simulink model "sampleModel106"  (R2022a)
settings: Solver=VariableStepAuto  StartTime=0.0  StopTime=10.0  RelTol=1e-3
undefined symbols (not defined in the file): DiscIntNeverNeededParam, magnitude, Newton, Raphson
libraries: simulink x379, slpidlib x89
(part 2 of 16)

== system sampleModel106/cfblk78/cfblk12 ==
  cfblk1 : Inport
  cfblk6 : Inport  Port=2
  Action Port : ActionPort  ActionPortLabel=else
  cfblk3 : ComplexToMagnitudeAngle
  cfblk4 : Subsystem
  cfblk5 : Subsystem
  cfblk8 : Delay
  cfblk9 : Delay
  cfblk2 : Outport
  cfblk7 : Outport  Port=2
  wires:
  cfblk6/1 -> cfblk5/1(cfblk1)
  cfblk1/1 -> cfblk3/1
  cfblk4/1(cfblk2) -> cfblk5/2(cfblk11)
  cfblk4/2(cfblk14) -> cfblk2/1
  cfblk5/3(cfblk13) -> cfblk7/1
  cfblk3/1 -> cfblk4/3(cfblk12)
  cfblk3/2 -> cfblk4/4(cfblk13)
  cfblk5/1(cfblk2) -> cfblk8/1
  cfblk8/1 -> cfblk4/1(cfblk1)
  cfblk5/2(cfblk12) -> cfblk9/1
  cfblk9/1 -> cfblk4/2(cfblk11)

== system sampleModel106/cfblk79/cfblk6 ==
  cfblk1 : Inport
  cfblk10 : Delay  SampleTime=1
  cfblk3 : Product
  cfblk4 : Squeeze
  cfblk5 : Product
  cfblk6 : Constant  Value=[-50724463.125212]  SampleTime=1
  cfblk7 : Constant  Value=[-745768619.596792]  SampleTime=1
  cfblk8 : Subsystem
  cfblk9 : Delay  SampleTime=1
  cfblk2 : Outport
  wires:
  cfblk4/1 -> cfblk2/1
  cfblk6/1 -> cfblk4/1
  cfblk7/1 -> cfblk3/1
  cfblk1/1 -> cfblk8/1(cfblk1)
  cfblk8/1(cfblk2) -> cfblk5/1
  cfblk8/2(cfblk9) -> cfblk3/2, cfblk5/2
  cfblk5/1 -> cfblk9/1
  cfblk9/1 -> cfblk8/3(cfblk8)
  cfblk3/1 -> cfblk10/1
  cfblk10/1 -> cfblk8/2(cfblk7)

== system sampleModel106/cfblk79/cfblk7 ==
  cfblk1 : Inport
  cfblk14 : Inport  Port=2
  cfblk15 : Inport  Port=3
  cfblk10 : Subsystem
  cfblk11 : Subsystem
  cfblk12 : Subsystem
  cfblk13 : Subsystem
  cfblk16 : Delay  SampleTime=1
  cfblk17 : Delay  SampleTime=1
  cfblk3 : DiscreteStateSpace
  cfblk4 : DiscreteZeroPole  Poles=[0 0.5]  Gain=1
  cfblk5 : simulink/Discrete/Tapped Delay  vinit=0.0  samptime=-1  NumDelays=1  DelayOrder=Oldest  includeCurrent=off
  cfblk6 : simulink/Math Operations/MinMax Running Resettable  Function=min  vinit=0.0
  cfblk7 : simulink/Math Operations/MinMax Running Resettable  Function=min  vinit=0.0
  cfblk8 : Constant  Value=[66779856.754441]  SampleTime=1
  cfblk9 : Constant  Value=[74672410.841103]  SampleTime=1
  cfblk2 : Outport
  wires:
  cfblk15/1 -> cfblk7/1
  cfblk11/1(cfblk2) -> cfblk5/1
  cfblk5/1 -> cfblk3/1
  cfblk13/1(cfblk2) -> cfblk2/1
  cfblk7/1 -> cfblk13/1(cfblk1)
  cfblk3/1 -> cfblk10/1(cfblk1)
  cfblk8/1 -> cfblk11/1(cfblk1)
  cfblk4/1 -> cfblk12/1(cfblk1)
  cfblk10/1(cfblk2) -> cfblk7/2
  cfblk1/1 -> cfblk6/2
  cfblk9/1 -> cfblk12/2(cfblk15)
  cfblk6/1 -> cfblk11/2(cfblk13)
  cfblk11/3(cfblk16) -> cfblk12/3(cfblk16)
  cfblk14/1 -> cfblk4/1
  cfblk11/2(cfblk15) -> cfblk16/1
  cfblk16/1 -> cfblk6/1
  cfblk12/1(cfblk2) -> cfblk17/1
  cfblk17/1 -> cfblk11/3(cfblk14)

== system sampleModel106/cfblk79/cfblk8 ==
  cfblk1 : Inport
  cfblk10 : Subsystem
  cfblk11 : Subsystem
  cfblk12 : Delay  SampleTime=1
  cfblk13 : Delay  SampleTime=1
  cfblk14 : Delay  SampleTime=1
  cfblk3 : Delay  DelayLengthSource=Input port  SampleTime=1
      settings: InputPortMap=u0,p1
  cfblk4 : slpidlib/PID Controller (2DOF)  Controller=PID  Form=Parallel  TimeDomain=Discrete-time  UseExternalTs=off  SampleTime=1  IntegratorMethod=Forward Euler  FilterMethod=Forward Euler  ControllerParametersSource=internal  P=1  I=1  UseKiTs=off  D=0  N=100  UseFilter=on  b=1  c=1  TunerSelectOption=Transfer Function Based (PID Tuner App)  InitialConditionSource=internal  InitialConditionForIntegrator=0  InitialConditionForFilter=0  DifferentiatorICPrevScaledInput=0  ExternalReset=none  TrackingMode=off  Kt=1  LimitOutput=off  SatLimitsSource=internal  UpperSaturationLimit=inf  LowerSaturationLimit=-inf  LinearizeAsGain=off  AntiWindupMode=none  Kb=1  POutMin=[]  POutMax=[]  IOutMin=[]  IOutMax=[]  DOutMin=[]  DOutMax=[]  NOutMin=[]  NOutMax=[]  bOutMin=[]  bOutMax=[]  cOutMin=[]  cOutMax=[]  SumOutMin=[]  SumOutMax=[]  SaturationOutMin=[]  SaturationOutMax=[]  PParamMin=[]  PParamMax=[]  IParamMin=[]  IParamMax=[]  DParamMin=[]  DParamMax=[]  NParamMin=[]  NParamMax=[]  bParamMin=[]  bParamMax=[]  cParamMin=[]  cParamMax=[]  KbParamMin=[]  KbParamMax=[]  KtParamMin=[]  KtParamMax=[]  KbOutMin=[]  KbOutMax=[]  KtOutMin=[]  KtOutMax=[]  IntegratorOutMin=[]  IntegratorOutMax=[]  FilterOutMin=[]  FilterOutMax=[]  SumI1OutMin=[]  SumI1OutMax=[]  SumI2OutMin=[]  SumI2OutMax=[]  SumI3OutMin=[]  SumI3OutMax=[]  SumI4OutMin=[]  SumI4OutMax=[]  SumDOutMin=[]  SumDOutMax=[]  Sum1OutMin=[]  Sum1OutMax=[]  Sum2OutMin=[]  Sum2OutMax=[]  Sum3OutMin=[]  Sum3OutMax=[]  DifferentiatorOutMin=[]  DifferentiatorOutMax=[]  FilterDiffOutCoefMin=[]  FilterDiffOutCoefMax=[]  ReciprocalOutMin=[]  ReciprocalOutMax=[]  SumDenOutMin=[]  SumDenOutMax=[]  SumNumOutMin=[]  SumNumOutMax=[]  DivideOutMin=[]  DivideOutMax=[]  UdiffTsProdOutMin=[]  UdiffTsProdOutMax=[]  NTsProdOutMin=[]  NTsProdOutMax=[]  UintegralTsProdOutMin=[]  UintegralTsProdOutMax=[]  UngainTsProdOutMin=[]  UngainTsProdOutMax=[]  IntegratorContinuousStateAttributes=''  IntegratorStateMustResolveToSignalObject=off  IntegratorRTWStateStorageClass=Auto  FilterContinuousStateAttributes=''  FilterStateMustResolveToSignalObject=off  FilterRTWStateStorageClass=Auto  ParallelPVariant=InternalParameters  IdealPVariant=Disabled  IVariant=InternalParameters  DVariant=InternalParameters  bVariant=InternalParameters  cVariant=InternalParameters  IntegratorVariant=Discrete  SatVariant=Disabled  AWVariant=Passthrough  PCopyVariant=Disabled  TRVariant=Disabled  FdbkBlocksVariant=Forward  IdealPFdbkVariant=Disabled  SatFdbkVariant=Disabled  DerivativeFilterVariant=ForwardEulerFilter  NVariant=InternalParameters  NCopyVariant=Disabled  FilterICVariant=InternalICsFilter  IntegratorICVariant=InternalICs  ExternalResetVariant=Disabled  TRSumVariant=Passthrough  SumFdbkVariant=Disabled  SumVariant=Sum_PID  TsampFilterVariant=InternalTs  TsampNgainVariant=Passthrough  TsampIntegralVariant=Passthrough  ExternalSaturationOutDataTypeStr=Inherit: Same as second input
      settings: SourceProductBaseCode=SL
  cfblk5 : DotProduct  OutDataTypeStr=Inherit: Inherit via internal rule
  cfblk6 : UnaryMinus
  cfblk7 : Constant  Value=[335459876.911431]  SampleTime=1
  cfblk8 : Constant  Value=[-968015926.513109]  SampleTime=1
  cfblk9 : Subsystem
  cfblk2 : Outport
  wires:
  cfblk8/1 -> cfblk10/1(cfblk1)
  cfblk10/1(cfblk2) -> cfblk6/1
  cfblk10/2(cfblk9) -> cfblk3/2
  cfblk9/1(cfblk2) -> cfblk11/1(cfblk1)
  cfblk11/1(cfblk2) -> cfblk4/1
  cfblk7/1 -> cfblk4/2
  cfblk1/1 -> cfblk2/1
  cfblk11/2(cfblk15) -> cfblk5/1
  cfblk6/1 -> cfblk9/1(cfblk1)
  cfblk10/3(cfblk10) -> cfblk5/2, cfblk11/2(cfblk14)
  cfblk3/1 -> cfblk9/3(cfblk11)
  cfblk4/1 -> cfblk12/1
  cfblk12/1 -> cfblk9/2(cfblk10)
  cfblk5/1 -> cfblk13/1
  cfblk13/1 -> cfblk3/1
  cfblk11/3(cfblk16) -> cfblk14/1
  cfblk14/1 -> cfblk9/4(cfblk12)

== system sampleModel106/cfblk80/cfblk10 ==
  cfblk1 : Inport
  cfblk14 : Inport  Port=2
  cfblk15 : Inport  Port=3
  cfblk10 : Subsystem
  cfblk11 : Subsystem
  cfblk12 : Subsystem
  cfblk13 : If  IfExpression=u1 >= 0  SampleTime=1
  cfblk16 : Subsystem  TreatAsAtomicUnit=on
  cfblk17 : Subsystem  TreatAsAtomicUnit=on
  cfblk18 : Delay  SampleTime=1
  cfblk19 : Delay  SampleTime=1
  cfblk3 : UnitDelay  HasFrameUpgradeWarning=on
  cfblk4 : Math  Operator=transpose
  cfblk5 : Product
  cfblk6 : Signum
  cfblk7 : Subsystem
  cfblk8 : Subsystem
  cfblk9 : Subsystem
  cfblk2 : Outport
  wires:
  cfblk3/1 -> cfblk4/1
  cfblk14/1 -> cfblk10/1(cfblk1), cfblk8/1(cfblk1), cfblk17/2(cfblk16)
  cfblk1/1 -> cfblk10/2(cfblk13)
  cfblk8/1(cfblk2) -> cfblk7/1(cfblk1)
  cfblk7/1(cfblk2) -> cfblk13/1
  cfblk5/1 -> cfblk11/1(cfblk1)
  cfblk17/1(cfblk2) -> cfblk12/1(cfblk1)
  cfblk17/2(cfblk17) -> cfblk3/1
  cfblk10/1(cfblk2) -> cfblk9/2(cfblk10)
  cfblk12/1(cfblk2) -> cfblk5/1
  cfblk12/2(cfblk10) -> cfblk6/1
  cfblk16/1(cfblk2) -> cfblk5/2
  cfblk12/3(cfblk11) -> cfblk11/2(cfblk15)
  cfblk6/1 -> cfblk2/1
  cfblk15/1 -> cfblk9/3(cfblk11)
  cfblk9/1(cfblk2) -> cfblk16/2(cfblk7)
  cfblk10/2(cfblk14) -> cfblk17/1(cfblk1)
  cfblk13/1 -> cfblk16/Action
  cfblk13/2 -> cfblk17/Action
  cfblk11/1(cfblk2) -> cfblk18/1
  cfblk18/1 -> cfblk9/1(cfblk1)
  cfblk4/1 -> cfblk19/1
  cfblk19/1 -> cfblk16/1(cfblk1)

== system sampleModel106/cfblk80/cfblk11 ==
  cfblk1 : Inport
  cfblk11 : Inport  Port=2
  cfblk12 : Inport  Port=3
  cfblk10 : Subsystem
  cfblk15 : Delay  SampleTime=1
  cfblk16 : Delay  SampleTime=1
  cfblk3 : UnitDelay  HasFrameUpgradeWarning=on
  cfblk4 : UnitDelay  HasFrameUpgradeWarning=on
  cfblk5 : Delay  DelayLengthSource=Input port  SampleTime=1
      settings: InputPortMap=u0,p1
  cfblk6 : Abs  SaturateOnIntegerOverflow=off
  cfblk7 : Abs  SaturateOnIntegerOverflow=off
  cfblk8 : Subsystem
  cfblk9 : Subsystem
  cfblk2 : Outport
  cfblk13 : Outport  Port=2
  cfblk14 : Outport  Port=3
  wires:
  cfblk7/1 -> cfblk4/1
  cfblk10/1(cfblk2) -> cfblk3/1, cfblk8/4(cfblk15)
  cfblk11/1 -> cfblk13/1, cfblk9/3(cfblk15)
  cfblk12/1 -> cfblk2/1
  cfblk1/1 -> cfblk9/1(cfblk1)
  cfblk4/1 -> cfblk8/1(cfblk1)
  cfblk3/1 -> cfblk7/1
  cfblk9/1(cfblk2) -> cfblk6/1
  cfblk6/1 -> cfblk14/1
  cfblk5/1 -> cfblk8/2(cfblk13), cfblk15/1
  cfblk9/2(cfblk16) -> cfblk5/2
  cfblk9/3(cfblk17) -> cfblk10/1(cfblk1), cfblk8/3(cfblk14)
  cfblk15/1 -> cfblk9/2(cfblk14)
  cfblk8/1(cfblk2) -> cfblk16/1
  cfblk16/1 -> cfblk5/1

== system sampleModel106/cfblk80/cfblk12 ==
  cfblk1 : Inport
  cfblk10 : Inport  Port=2
  cfblk11 : Inport  Port=3
  cfblk13 : Delay  SampleTime=1
  cfblk3 : simulink/Math Operations/MinMax Running Resettable  Function=min  vinit=0.0
  cfblk4 : simulink/Math Operations/MinMax Running Resettable  Function=min  vinit=0.0
  cfblk5 : Constant  Value=[977677055.590889]  SampleTime=1
  cfblk6 : Constant  Value=[-64225626.397108]  SampleTime=1
  cfblk7 : Constant  Value=[-755451288.420639]  SampleTime=1
  cfblk8 : Constant  Value=[-818937205.633430]  SampleTime=1
  cfblk9 : Subsystem
  cfblk2 : Outport
  cfblk12 : Outport  Port=2
  wires:
  cfblk5/1 -> cfblk12/1
  cfblk10/1 -> cfblk3/1
  cfblk1/1 -> cfblk2/1
  cfblk4/1 -> cfblk9/1(cfblk1)
  cfblk11/1 -> cfblk3/2
  cfblk8/1 -> cfblk4/2
  cfblk9/1(cfblk2) -> cfblk13/1
  cfblk13/1 -> cfblk4/1

== system sampleModel106/cfblk80/cfblk8 ==
  cfblk1 : Inport
  cfblk9 : Inport  Port=2
  cfblk10 : Inport  Port=3
  cfblk11 : Inport  Port=4
  cfblk3 : simulink/Discrete/Transfer Fcn First Order  PoleZ=0.95  ICPrevOutput=0.0  DoSatur=off
  cfblk4 : Constant  Value=[816794916.066360]  SampleTime=1
  cfblk5 : Constant  Value=[815613005.147232]  SampleTime=1
  cfblk6 : Constant  Value=[-885196451.033393]  SampleTime=1
  cfblk7 : Subsystem
  cfblk8 : Subsystem
  cfblk2 : Outport
  wires:
  cfblk5/1 -> cfblk3/1
  cfblk6/1 -> cfblk7/1(cfblk1)
  cfblk1/1 -> cfblk7/2(cfblk7)
  cfblk10/1 -> cfblk2/1
  cfblk9/1 -> cfblk8/1(cfblk1)

== system sampleModel106/cfblk80/cfblk9 ==
  cfblk1 : Inport
  cfblk8 : Inport  Port=2
  cfblk11 : Subsystem  TreatAsAtomicUnit=on
  cfblk12 : Subsystem  TreatAsAtomicUnit=on
  cfblk13 : Delay  SampleTime=1
  cfblk3 : simulink/Discrete/Transfer Fcn Real Zero  ZeroZ=0.75  ICPrevInput=0.0  DoSatur=off
      settings: SourceProductBaseCode=SL
  cfblk4 : Trigonometry
  cfblk5 : Sin  TimeSource=Use external signal  SampleTime=0
  cfblk6 : Subsystem
  cfblk7 : If  IfExpression=u1 >= 0  SampleTime=1
  cfblk2 : Outport
  cfblk9 : Outport  Port=2
  cfblk10 : Outport  Port=3
  wires:
  cfblk5/1 -> cfblk3/1, cfblk9/1
  cfblk11/1(cfblk2) -> cfblk6/1(cfblk1)
  cfblk1/1 -> cfblk7/1, cfblk5/1
  cfblk12/1(cfblk2) -> cfblk6/2(cfblk15)
  cfblk8/1 -> cfblk6/3(cfblk16)
  cfblk11/2(cfblk11) -> cfblk12/1(cfblk1)
  cfblk6/1(cfblk2) -> cfblk2/1, cfblk13/1
  cfblk3/1 -> cfblk4/1
  cfblk4/1 -> cfblk10/1, cfblk11/1(cfblk1)
  cfblk7/1 -> cfblk11/Action
  cfblk7/2 -> cfblk12/Action
  cfblk13/1 -> cfblk11/2(cfblk10)

== system sampleModel106/cfblk81/cfblk8 ==
  cfblk1 : Inport
  cfblk7 : Inport  Port=2
  cfblk8 : Inport  Port=3
  cfblk9 : Inport  Port=4
  cfblk10 : Inport  Port=5
  cfblk13 : Delay  SampleTime=1
  cfblk3 : Constant  Value=[-561952137.988707]  SampleTime=1
  cfblk4 : Subsystem
  cfblk5 : Subsystem
  cfblk6 : Subsystem
  cfblk2 : Outport
  cfblk11 : Outport  Port=2
  cfblk12 : Outport  Port=3
  wires:
  cfblk7/1 -> cfblk5/1(cfblk1)
  cfblk1/1 -> cfblk12/1
  cfblk10/1 -> cfblk2/1
  cfblk9/1 -> cfblk5/2(cfblk9), cfblk6/4(cfblk14)
  cfblk3/1 -> cfblk4/1(cfblk1), cfblk6/2(cfblk12)
  cfblk8/1 -> cfblk11/1
  cfblk4/1(cfblk2) -> cfblk6/1(cfblk1)
  cfblk5/1(cfblk2) -> cfblk4/3(cfblk7), cfblk6/3(cfblk13)
  cfblk6/1(cfblk2) -> cfblk13/1
  cfblk13/1 -> cfblk4/2(cfblk6)

== system sampleModel106/cfblk82/cfblk7 ==
  cfblk1 : Inport
  cfblk10 : Inport  Port=2
  cfblk11 : Inport  Port=3
  cfblk12 : Subsystem  TreatAsAtomicUnit=on
  cfblk13 : Subsystem  TreatAsAtomicUnit=on
  cfblk{14..21} (8 alike) : Delay  SampleTime=1
  cfblk3 : PermuteDimensions
  cfblk4 : Sum  Inputs=|++
  cfblk5 : Product  Inputs=**
  cfblk6 : Subsystem
  cfblk7 : Subsystem
  cfblk8 : Subsystem
  cfblk9 : If  IfExpression=u1 >= 0  SampleTime=1
  cfblk2 : Outport
  wires:
  cfblk7/1(cfblk2) -> cfblk4/1
  cfblk1/1 -> cfblk9/1, cfblk6/3(cfblk13)
  cfblk3/1 -> cfblk2/1
  cfblk8/1(cfblk2) -> cfblk3/1
  cfblk10/1 -> cfblk4/2, cfblk8/2(cfblk15)
  cfblk11/1 -> cfblk6/1(cfblk1)
  cfblk12/1(cfblk2) -> cfblk7/1(cfblk1)
  cfblk5/1 -> cfblk6/2(cfblk12), cfblk18/1, cfblk20/1
  cfblk13/2(cfblk9) -> cfblk8/1(cfblk1)
  cfblk8/3(cfblk17) -> cfblk5/1, cfblk5/2, cfblk17/1, cfblk21/1
  cfblk9/1 -> cfblk12/Action
  cfblk9/2 -> cfblk13/Action
  cfblk4/1 -> cfblk14/1
  cfblk14/1 -> cfblk13/2(cfblk7)
  cfblk13/1(cfblk2) -> cfblk15/1
  cfblk15/1 -> cfblk12/1(cfblk1)
  cfblk8/2(cfblk16) -> cfblk16/1
  cfblk16/1 -> cfblk7/2(cfblk14)
  cfblk17/1 -> cfblk12/2(cfblk8)
  cfblk18/1 -> cfblk13/3(cfblk8)
  cfblk6/1(cfblk2) -> cfblk19/1
  cfblk19/1 -> cfblk13/1(cfblk1)
  cfblk20/1 -> cfblk7/3(cfblk15)
  cfblk21/1 -> cfblk7/4(cfblk16)

== system sampleModel106/cfblk82/cfblk8 ==
  cfblk1 : Inport
  cfblk11 : Inport  Port=2
  cfblk10 : Subsystem
  cfblk3 : Assignment  DiagnosticForDimensions=Warning  IndexOptions=Index vector (dialog)  Indices=1  OutputSizes=1
  cfblk4 : Sum  Inputs=+-
  cfblk5 : simulink/Math Operations/Slider Gain  gain=1  low=0  high=2
  cfblk6 : Trigonometry
  cfblk7 : Constant  Value=[107354283.028272]  SampleTime=1
  cfblk8 : Constant  Value=[597705512.907011]  SampleTime=1
  cfblk9 : Constant  Value=[41432939.561174]  SampleTime=1
  cfblk2 : Outport
  wires:
  cfblk7/1 -> cfblk5/1
  cfblk8/1 -> cfblk3/1
  cfblk5/1 -> cfblk2/1
  cfblk10/1(cfblk2) -> cfblk4/1
  cfblk9/1 -> cfblk6/1
  cfblk6/1 -> cfblk3/2
  cfblk11/1 -> cfblk4/2
  cfblk3/1 -> cfblk10/1(cfblk1)

== system sampleModel106/cfblk83/cfblk11 ==
  cfblk1 : Inport
  cfblk12 : Inport  Port=2
  cfblk13 : Inport  Port=3
  cfblk10 : Subsystem
  cfblk11 : Subsystem
  cfblk{16..19} (4 alike) : Delay  SampleTime=1
  cfblk3 : Sum  Inputs=|++
  cfblk4 : Bias  Bias=[-264366451.714960]  SaturateOnIntegerOverflow=off
  cfblk5 : Squeeze
  cfblk6 : Constant  Value=[-682121101.648603]  SampleTime=1
  cfblk7 : Constant  Value=[950887714.893864]  SampleTime=1
  cfblk8 : Subsystem
  cfblk9 : Subsystem
  cfblk2 : Outport
  cfblk14 : Outport  Port=2
  cfblk15 : Outport  Port=3
  wires:
  cfblk5/1 -> cfblk11/1(cfblk1)
  cfblk10/1(cfblk2) -> cfblk11/2(cfblk6)
  cfblk12/1 -> cfblk4/1
  cfblk7/1 -> cfblk5/1
  cfblk8/1(cfblk2) -> cfblk9/1(cfblk1)
  cfblk13/1 -> cfblk14/1
  cfblk6/1 -> cfblk8/1(cfblk1)
  cfblk3/1 -> cfblk9/2(cfblk10)
  cfblk9/1(cfblk2) -> cfblk10/1(cfblk1)
  cfblk4/1 -> cfblk8/2(cfblk10)
  cfblk9/2(cfblk12) -> cfblk15/1
  cfblk10/2(cfblk13) -> cfblk2/1
  cfblk11/1(cfblk2) -> cfblk16/1
  cfblk16/1 -> cfblk3/1
  cfblk11/2(cfblk7) -> cfblk17/1
  cfblk17/1 -> cfblk9/3(cfblk11)
  cfblk11/3(cfblk8) -> cfblk18/1
  cfblk18/1 -> cfblk10/2(cfblk12)
  cfblk9/3(cfblk13) -> cfblk19/1
  cfblk19/1 -> cfblk3/2

== system sampleModel106/cfblk83/cfblk12 ==
  cfblk1 : Inport
  cfblk10 : Constant  Value=[-740621265.953147]  SampleTime=1
  cfblk11 : Subsystem
  cfblk12 : Subsystem
  cfblk13 : Subsystem
  cfblk14 : Delay  SampleTime=1
  cfblk15 : Delay  SampleTime=1
  cfblk3 : DiscreteStateSpace
  cfblk4 : Sqrt  Operator=rSqrt  AlgorithmType=Newton-Raphson
  cfblk5 : Trigonometry
  cfblk6 : Sum  Inputs=+-
  cfblk7 : ComplexToMagnitudeAngle
  cfblk8 : Sin  TimeSource=Use external signal  SampleTime=0
  cfblk9 : Constant  Value=[-272360660.039801]  SampleTime=1
  cfblk2 : Outport
  wires:
  cfblk4/1 -> cfblk13/1(cfblk1)
  cfblk11/1(cfblk2) -> cfblk4/1
  cfblk3/1 -> cfblk2/1
  cfblk7/1 -> cfblk13/2(cfblk11)
  cfblk6/1 -> cfblk12/1(cfblk1)
  cfblk1/1 -> cfblk8/1
  cfblk12/1(cfblk2) -> cfblk3/1
  cfblk9/1 -> cfblk12/2(cfblk12)
  cfblk13/1(cfblk2) -> cfblk5/1
  cfblk13/2(cfblk12) -> cfblk6/2
  cfblk10/1 -> cfblk7/1, cfblk11/4(cfblk8)
  cfblk8/1 -> cfblk11/2(cfblk6)
  cfblk7/2 -> cfblk11/3(cfblk7)
  cfblk5/1 -> cfblk14/1
  cfblk14/1 -> cfblk11/1(cfblk1)
  cfblk12/2(cfblk13) -> cfblk15/1
  cfblk15/1 -> cfblk6/1

== system sampleModel106/cfblk83/cfblk13 ==
  cfblk1 : Inport
  cfblk14 : Inport  Port=2
  cfblk15 : Inport  Port=3
  cfblk16 : Inport  Port=4
  cfblk10 : Constant  Value=[-629799726.415625]  SampleTime=1
  cfblk11 : Subsystem
  cfblk12 : Subsystem
  cfblk13 : Subsystem
  cfblk18 : Delay  SampleTime=1
  cfblk19 : Delay  SampleTime=1
  cfblk3 : Delay  ShowEnablePort=on  SampleTime=1
      settings: InputPortMap=u0,e6
  cfblk4 : Sum  Inputs=|++
  cfblk5 : ComplexToRealImag
  cfblk6 : Product
  cfblk7 : simulink/Math Operations/Slider Gain  gain=1  low=0  high=2
  cfblk8 : Assignment  DiagnosticForDimensions=Warning  IndexOptions=Index vector (dialog)  Indices=1  OutputSizes=1
  cfblk9 : PermuteDimensions
  cfblk2 : Outport
  cfblk17 : Outport  Port=2
  wires:
  cfblk5/1 -> cfblk13/1(cfblk1)
  cfblk12/1(cfblk2) -> cfblk9/1
  cfblk6/1 -> cfblk17/1
  cfblk1/1 -> cfblk2/1
  cfblk16/1 -> cfblk4/1
  cfblk11/1(cfblk2) -> cfblk4/2
  cfblk7/1 -> cfblk8/1
  cfblk8/1 -> cfblk5/1
  cfblk4/1 -> cfblk6/1
  cfblk9/1 -> cfblk7/1
  cfblk10/1 -> cfblk8/2
  cfblk15/1 -> cfblk13/2(cfblk10)
  cfblk13/1(cfblk2) -> cfblk6/2
  cfblk14/1 -> cfblk11/1(cfblk1)
  cfblk3/1 -> cfblk12/1(cfblk1)
  cfblk5/2 -> cfblk11/2(cfblk10)
  cfblk13/2(cfblk11) -> cfblk18/1
  cfblk18/1 -> cfblk3/1
  cfblk13/3(cfblk12) -> cfblk19/1
  cfblk19/1 -> cfblk3/2

== system sampleModel106/cfblk84/cfblk10 ==
  cfblk1 : Inport
  Action Port : ActionPort  ActionPortLabel=else
  cfblk10 : Subsystem
  cfblk{11..14} (4 alike) : Delay
  cfblk3 : Gain  Gain=[473633439.409636]
  cfblk4 : Product  Inputs=**
  cfblk5 : ComplexToRealImag
  cfblk6 : Constant  Value=[-365380379.420493]  SampleTime=1
  cfblk7 : Constant  Value=[556784110.226366]  SampleTime=1
  cfblk8 : Subsystem
  cfblk9 : Subsystem
  cfblk2 : Outport
  wires:
  cfblk6/1 -> cfblk3/1
  cfblk3/1 -> cfblk9/1(cfblk1), cfblk9/3(cfblk8)
  cfblk5/1 -> cfblk4/1
  cfblk10/1(cfblk2) -> cfblk9/2(cfblk7)
  cfblk1/1 -> cfblk5/1, cfblk8/5(cfblk12)
  cfblk5/2 -> cfblk8/1(cfblk1)
  cfblk7/1 -> cfblk2/1
  cfblk4/1 -> cfblk10/1(cfblk1)
  cfblk10/2(cfblk15) -> cfblk8/2(cfblk9)
  cfblk9/4(cfblk11) -> cfblk8/3(cfblk10)
  cfblk10/3(cfblk16) -> cfblk8/4(cfblk11)
  cfblk9/1(cfblk2) -> cfblk11/1
  cfblk11/1 -> cfblk4/2
  cfblk9/2(cfblk9) -> cfblk12/1
  cfblk12/1 -> cfblk10/3(cfblk13)
  cfblk9/3(cfblk10) -> cfblk13/1
  cfblk13/1 -> cfblk10/4(cfblk14)
  cfblk8/1(cfblk2) -> cfblk14/1
  cfblk14/1 -> cfblk10/2(cfblk12)

== system sampleModel106/cfblk84/cfblk5 ==
  cfblk1 : Inport
  cfblk15 : Inport  Port=2
  cfblk10 : Constant  Value=[615411436.639995]  SampleTime=1
  cfblk11 : Constant  Value=[182127342.306380]  SampleTime=1
  cfblk12 : Constant  Value=[-234776803.757724]  SampleTime=1
  cfblk13 : Subsystem
  cfblk14 : Subsystem
  cfblk3 : UnitDelay  HasFrameUpgradeWarning=on
  cfblk4 : DiscreteTransferFcn  SampleTime=1
  cfblk5 : UnitDelay  HasFrameUpgradeWarning=on
  cfblk6 : Signum
  cfblk7 : UnaryMinus
  cfblk8 : Sum  Inputs=+-
  cfblk9 : Product
  cfblk2 : Outport
  cfblk16 : Outport  Port=2
  cfblk17 : Outport  Port=3
  wires:
  cfblk4/1 -> cfblk5/1
  cfblk10/1 -> cfblk6/1
  cfblk1/1 -> cfblk14/1(cfblk1)
  cfblk14/1(cfblk2) -> cfblk4/1
  cfblk5/1 -> cfblk16/1, cfblk13/2(cfblk15)
  cfblk7/1 -> cfblk17/1
  cfblk11/1 -> cfblk3/1
  cfblk6/1 -> cfblk2/1
  cfblk8/1 -> cfblk13/1(cfblk1)
  cfblk3/1 -> cfblk9/1, cfblk13/4(cfblk17)
  cfblk15/1 -> cfblk8/1
  cfblk14/2(cfblk14) -> cfblk7/1
  cfblk9/1 -> cfblk8/2, cfblk13/3(cfblk16)
  cfblk12/1 -> cfblk9/2

== system sampleModel106/cfblk84/cfblk6 ==
  cfblk1 : Inport
  cfblk8 : Inport  Port=2
  cfblk9 : Inport  Port=3
  cfblk10 : Inport  Port=4
  cfblk11 : Inport  Port=5
  cfblk12 : Inport  Port=6
  cfblk3 : Sqrt  Operator=rSqrt  AlgorithmType=Newton-Raphson
  cfblk4 : Abs  SaturateOnIntegerOverflow=off
  cfblk5 : Subsystem
  cfblk6 : Subsystem
  cfblk7 : Subsystem
  cfblk2 : Outport
  wires:
  cfblk7/1(cfblk2) -> cfblk2/1
  cfblk11/1 -> cfblk5/1(cfblk1)
  cfblk6/1(cfblk2) -> cfblk3/1
  cfblk9/1 -> cfblk6/1(cfblk1)
  cfblk10/1 -> cfblk4/1
  cfblk4/1 -> cfblk5/2(cfblk13)
  cfblk6/2(cfblk14) -> cfblk7/1(cfblk1)
  cfblk1/1 -> cfblk7/2(cfblk12)
  cfblk3/1 -> cfblk5/3(cfblk14)
  cfblk12/1 -> cfblk5/4(cfblk15)
  cfblk8/1 -> cfblk5/5(cfblk16)

== system sampleModel106/cfblk84/cfblk9 ==
  cfblk1 : Inport
  cfblk14 : Inport  Port=2
  Action Port : ActionPort  ActionPortLabel=if(u1 >= 0)
  cfblk10 : Subsystem
  cfblk11 : Subsystem
  cfblk12 : Subsystem
  cfblk13 : Subsystem
  cfblk16 : Delay
  cfblk3 : slpidlib/PID Controller  Controller=PID  Form=Parallel  TimeDomain=Discrete-time  UseExternalTs=off  SampleTime=-1  IntegratorMethod=Forward Euler  FilterMethod=Forward Euler  ControllerParametersSource=internal  P=1  I=1  UseKiTs=off  D=0  N=100  UseFilter=on  TunerSelectOption=Transfer Function Based (PID Tuner App)  InitialConditionSource=internal  InitialConditionForIntegrator=0  InitialConditionForFilter=0  DifferentiatorICPrevScaledInput=0  ExternalReset=none  TrackingMode=off  Kt=1  LimitOutput=off  SatLimitsSource=internal  UpperSaturationLimit=inf  LowerSaturationLimit=-inf  LinearizeAsGain=off  AntiWindupMode=none  Kb=1  POutMin=[]  POutMax=[]  IOutMin=[]  IOutMax=[]  DOutMin=[]  DOutMax=[]  NOutMin=[]  NOutMax=[]  SumOutMin=[]  SumOutMax=[]  SaturationOutMin=[]  SaturationOutMax=[]  PParamMin=[]  PParamMax=[]  IParamMin=[]  IParamMax=[]  DParamMin=[]  DParamMax=[]  NParamMin=[]  NParamMax=[]  KbParamMin=[]  KbParamMax=[]  KtParamMin=[]  KtParamMax=[]  KbOutMin=[]  KbOutMax=[]  KtOutMin=[]  KtOutMax=[]  IntegratorOutMin=[]  IntegratorOutMax=[]  FilterOutMin=[]  FilterOutMax=[]  SumI1OutMin=[]  SumI1OutMax=[]  SumI2OutMin=[]  SumI2OutMax=[]  SumI3OutMin=[]  SumI3OutMax=[]  SumI4OutMin=[]  SumI4OutMax=[]  SumDOutMin=[]  SumDOutMax=[]  DifferentiatorOutMin=[]  DifferentiatorOutMax=[]  FilterDiffOutCoefMin=[]  FilterDiffOutCoefMax=[]  ReciprocalOutMin=[]  ReciprocalOutMax=[]  SumDenOutMin=[]  SumDenOutMax=[]  SumNumOutMin=[]  SumNumOutMax=[]  DivideOutMin=[]  DivideOutMax=[]  UdiffTsProdOutMin=[]  UdiffTsProdOutMax=[]  NTsProdOutMin=[]  NTsProdOutMax=[]  UintegralTsProdOutMin=[]  UintegralTsProdOutMax=[]  UngainTsProdOutMin=[]  UngainTsProdOutMax=[]  IntegratorContinuousStateAttributes=''  IntegratorStateMustResolveToSignalObject=off  IntegratorRTWStateStorageClass=Auto  FilterContinuousStateAttributes=''  FilterStateMustResolveToSignalObject=off  FilterRTWStateStorageClass=Auto  ParallelPVariant=InternalParameters  IdealPVariant=Disabled  IVariant=InternalParameters  DVariant=InternalParameters  IntegratorVariant=Discrete  SatVariant=Disabled  AWVariant=Passthrough  PCopyVariant=Disabled  TRVariant=Disabled  FdbkBlocksVariant=Forward  IdealPFdbkVariant=Disabled  SatFdbkVariant=Disabled  DerivativeFilterVariant=ForwardEulerFilter  NVariant=InternalParameters  NCopyVariant=Disabled  FilterICVariant=InternalICsFilter  IntegratorICVariant=InternalICs  ExternalResetVariant=Disabled  TRSumVariant=Passthrough  SumFdbkVariant=Disabled  SumVariant=Sum_PID  TsampFilterVariant=InternalTs  TsampNgainVariant=Passthrough  TsampIntegralVariant=Passthrough  ExternalSaturationOutDataTypeStr=Inherit: Same as second input  aMode=0
  cfblk4 : simulink/Math Operations/Slider Gain  gain=1  low=0  high=2
  cfblk5 : Rounding
  cfblk6 : Abs  SaturateOnIntegerOverflow=off
  cfblk7 : Constant  Value=[-771466192.813952]  SampleTime=1
  cfblk8 : Constant  Value=[252961666.133108]  SampleTime=1
  cfblk9 : Constant  Value=[497467020.643406]  SampleTime=1
  cfblk2 : Outport
  cfblk15 : Outport  Port=2
  wires:
  cfblk8/1 -> cfblk3/1
  cfblk11/1(cfblk2) -> cfblk15/1
  cfblk11/2(cfblk14) -> cfblk2/1
  cfblk10/1(cfblk2) -> cfblk5/1
  cfblk5/1 -> cfblk6/1
  cfblk3/1 -> cfblk4/1
  cfblk12/1(cfblk2) -> cfblk13/1(cfblk1)
  cfblk6/1 -> cfblk12/1(cfblk1)
  cfblk14/1 -> cfblk12/2(cfblk7)
  cfblk11/3(cfblk15) -> cfblk10/1(cfblk1)
  cfblk7/1 -> cfblk13/2(cfblk12)
  cfblk4/1 -> cfblk10/2(cfblk11)
  cfblk1/1 -> cfblk11/1(cfblk1)
  cfblk9/1 -> cfblk13/3(cfblk13)
  cfblk13/1(cfblk2) -> cfblk16/1
  cfblk16/1 -> cfblk11/2(cfblk13)

== system sampleModel106/cfblk86/cfblk10 ==
  cfblk1 : Inport
  cfblk14 : Inport  Port=2
  cfblk15 : Inport  Port=3
  cfblk16 : Inport  Port=4
  cfblk10 : Subsystem
  cfblk11 : Subsystem
  cfblk12 : Subsystem
  cfblk13 : Subsystem
  cfblk17 : Delay
  cfblk18 : Delay
  cfblk3 : simulink/Discrete/Difference  ICPrevInput=0.0  OutMin=[]  OutMax=[]  OutDataTypeStr=Inherit: Inherit via back propagation  OutDataType=fixdt(1, 16)  OutScaling=2^-10  DoSatur=off
  cfblk4 : simulink/Math Operations/Slider Gain  gain=1  low=0  high=2
  cfblk5 : MinMax  Function=max
  cfblk6 : Sum  Inputs=--
  cfblk7 : Product  Inputs=**
  cfblk8 : Constant  Value=[347377700.754790]  SampleTime=1
  cfblk9 : Subsystem
  cfblk2 : Outport
  wires:
  cfblk10/1(cfblk2) -> cfblk7/1
  cfblk16/1 -> cfblk12/1(cfblk1), cfblk12/4(cfblk9)
  cfblk12/1(cfblk2) -> cfblk6/1
  cfblk13/1(cfblk2) -> cfblk9/1(cfblk1)
  cfblk13/2(cfblk14) -> cfblk9/2(cfblk10)
  cfblk15/1 -> cfblk7/2
  cfblk14/1 -> cfblk5/1, cfblk13/2(cfblk12)
  cfblk4/1 -> cfblk11/1(cfblk1)
  cfblk5/1 -> cfblk3/1
  cfblk3/1 -> cfblk6/2
  cfblk8/1 -> cfblk11/2(cfblk10)
  cfblk11/1(cfblk2) -> cfblk2/1
  cfblk1/1 -> cfblk12/2(cfblk7)
  cfblk6/1 -> cfblk4/1
  cfblk12/2(cfblk10) -> cfblk10/2(cfblk7), cfblk11/3(cfblk11)
  cfblk11/2(cfblk12) -> cfblk13/1(cfblk1), cfblk13/3(cfblk13)
  cfblk9/1(cfblk2) -> cfblk17/1
  cfblk17/1 -> cfblk12/3(cfblk8)
  cfblk7/1 -> cfblk18/1
  cfblk18/1 -> cfblk10/1(cfblk1)

== system sampleModel106/cfblk86/cfblk11 ==
  cfblk1 : Inport
  cfblk3 : simulink/Discrete/Transfer Fcn Real Zero  ZeroZ=0.75  ICPrevInput=0.0  DoSatur=off
      settings: SourceProductBaseCode=SL
  cfblk4 : Sqrt
  cfblk5 : Constant  Value=[-201211534.488283]  SampleTime=1
  cfblk6 : Constant  Value=[-198237638.731212]  SampleTime=1
  cfblk7 : Subsystem
  cfblk8 : Subsystem
  cfblk9 : Delay
  cfblk2 : Outport
  wires:
  cfblk5/1 -> cfblk2/1
  cfblk8/1(cfblk2) -> cfblk4/1
  cfblk1/1 -> cfblk8/1(cfblk1)
  cfblk7/1(cfblk2) -> cfblk3/1
  cfblk6/1 -> cfblk7/1(cfblk1)
  cfblk3/1 -> cfblk8/3(cfblk14)
  cfblk4/1 -> cfblk9/1
  cfblk9/1 -> cfblk8/2(cfblk13)

== system sampleModel106/cfblk86/cfblk12 ==
  cfblk1 : Inport
  cfblk12 : Inport  Port=2
  cfblk10 : Subsystem
  cfblk11 : Subsystem
  cfblk{13..17} (5 alike) : Delay
  cfblk3 : Delay  ShowEnablePort=on
      settings: InputPortMap=u0,e6
  cfblk4 : Reshape
  cfblk5 : Constant  Value=[-767740041.430021]  SampleTime=1
  cfblk6 : Subsystem
  cfblk7 : Subsystem
  cfblk8 : Subsystem
  cfblk9 : Subsystem
  cfblk2 : Outport
  wires:
  cfblk12/1 -> cfblk2/1
  cfblk3/1 -> cfblk11/1(cfblk1)
  cfblk1/1 -> cfblk7/2(cfblk9), cfblk7/3(cfblk10)
  cfblk6/1(cfblk2) -> cfblk8/1(cfblk1)
  cfblk7/1(cfblk2) -> cfblk9/2(cfblk8)
  cfblk6/2(cfblk12) -> cfblk8/2(cfblk11)
  cfblk7/2(cfblk14) -> cfblk8/3(cfblk12)
  cfblk4/1 -> cfblk11/2(cfblk13)
  cfblk5/1 -> cfblk6/1(cfblk1)
  cfblk10/1(cfblk2) -> cfblk6/2(cfblk10)
  cfblk10/2(cfblk16) -> cfblk6/3(cfblk11), cfblk15/1, cfblk16/1, cfblk17/1
  cfblk9/1(cfblk2) -> cfblk10/1(cfblk1)
  cfblk6/3(cfblk13) -> cfblk4/1, cfblk3/1, cfblk3/2, cfblk11/3(cfblk14)
  cfblk8/1(cfblk2) -> cfblk13/1
  cfblk13/1 -> cfblk9/1(cfblk1)
  cfblk11/1(cfblk2) -> cfblk14/1
  cfblk14/1 -> cfblk7/1(cfblk1)
  cfblk15/1 -> cfblk7/4(cfblk11)
  cfblk16/1 -> cfblk7/5(cfblk12)
  cfblk17/1 -> cfblk7/6(cfblk13)

== system sampleModel106/cfblk86/cfblk13 ==
  cfblk1 : Inport
  cfblk{8..11} (4 alike) : Delay
  cfblk3 : Polyval  Coefs=[ +2.081618890e-019, -1.441693666e-014, +4.719686976e-010, -8.536869453e-006, +1.621573104e-001, -8.087801117e+001 ]
  cfblk4 : MinMax  Inputs=3
  cfblk5 : Subsystem
  cfblk6 : Subsystem
  cfblk7 : Subsystem
  cfblk2 : Outport
  wires:
  cfblk3/1 -> cfblk4/2, cfblk7/3(cfblk8), cfblk4/3, cfblk8/1
  cfblk7/1(cfblk2) -> cfblk4/1, cfblk10/1
  cfblk5/1(cfblk2) -> cfblk3/1
  cfblk5/2(cfblk14) -> cfblk7/1(cfblk1), cfblk7/2(cfblk7), cfblk11/1
  cfblk6/1(cfblk2) -> cfblk2/1, cfblk5/2(cfblk13)
  cfblk1/1 -> cfblk6/3(cfblk8)
  cfblk8/1 -> cfblk6/1(cfblk1)
  cfblk4/1 -> cfblk9/1
  cfblk9/1 -> cfblk5/1(cfblk1)
  cfblk10/1 -> cfblk6/2(cfblk7)
  cfblk11/1 -> cfblk6/4(cfblk9)

== system sampleModel106/cfblk86/cfblk9 ==
  cfblk1 : Inport
  cfblk9 : Inport  Port=2
  cfblk10 : Inport  Port=3
  cfblk11 : Inport  Port=4
  cfblk3 : simulink/Discrete/Transfer Fcn Lead or Lag  PoleZ=0.95  ZeroZ=0.75  ICPrevOutput=0.0  ICPrevInput=0.0  DoSatur=off
      settings: SourceProductBaseCode=SL
  cfblk4 : Delay  DelayLengthSource=Input port
      settings: InputPortMap=u0,p1
  cfblk5 : Product  Inputs=**
  cfblk6 : Constant  Value=[-414962038.903637]  SampleTime=1
  cfblk7 : Constant  Value=[-45204893.637828]  SampleTime=1
  cfblk8 : Subsystem
  cfblk2 : Outport
  cfblk12 : Outport  Port=2
  wires:
  cfblk8/1(cfblk2) -> cfblk3/1
  cfblk7/1 -> cfblk2/1
  cfblk11/1 -> cfblk8/1(cfblk1)
  cfblk9/1 -> cfblk5/1
  cfblk5/1 -> cfblk4/1
  cfblk6/1 -> cfblk4/2
  cfblk10/1 -> cfblk12/1
  cfblk1/1 -> cfblk5/2

== system sampleModel106/cfblk87/cfblk7 ==
  cfblk1 : Inport
  cfblk12 : Inport  Port=2
  cfblk13 : Inport  Port=3
  cfblk10 : Subsystem
  cfblk11 : Subsystem
  cfblk16 : Delay
  cfblk3 : slpidlib/PID Controller (2DOF)  Controller=PID  Form=Parallel  TimeDomain=Discrete-time  UseExternalTs=off  SampleTime=-1  IntegratorMethod=Forward Euler  FilterMethod=Forward Euler  ControllerParametersSource=internal  P=1  I=1  UseKiTs=off  D=0  N=100  UseFilter=on  b=1  c=1  TunerSelectOption=Transfer Function Based (PID Tuner App)  InitialConditionSource=internal  InitialConditionForIntegrator=0  InitialConditionForFilter=0  DifferentiatorICPrevScaledInput=0  ExternalReset=none  TrackingMode=off  Kt=1  LimitOutput=off  SatLimitsSource=internal  UpperSaturationLimit=inf  LowerSaturationLimit=-inf  LinearizeAsGain=off  AntiWindupMode=none  Kb=1  POutMin=[]  POutMax=[]  IOutMin=[]  IOutMax=[]  DOutMin=[]  DOutMax=[]  NOutMin=[]  NOutMax=[]  bOutMin=[]  bOutMax=[]  cOutMin=[]  cOutMax=[]  SumOutMin=[]  SumOutMax=[]  SaturationOutMin=[]  SaturationOutMax=[]  PParamMin=[]  PParamMax=[]  IParamMin=[]  IParamMax=[]  DParamMin=[]  DParamMax=[]  NParamMin=[]  NParamMax=[]  bParamMin=[]  bParamMax=[]  cParamMin=[]  cParamMax=[]  KbParamMin=[]  KbParamMax=[]  KtParamMin=[]  KtParamMax=[]  KbOutMin=[]  KbOutMax=[]  KtOutMin=[]  KtOutMax=[]  IntegratorOutMin=[]  IntegratorOutMax=[]  FilterOutMin=[]  FilterOutMax=[]  SumI1OutMin=[]  SumI1OutMax=[]  SumI2OutMin=[]  SumI2OutMax=[]  SumI3OutMin=[]  SumI3OutMax=[]  SumI4OutMin=[]  SumI4OutMax=[]  SumDOutMin=[]  SumDOutMax=[]  Sum1OutMin=[]  Sum1OutMax=[]  Sum2OutMin=[]  Sum2OutMax=[]  Sum3OutMin=[]  Sum3OutMax=[]  DifferentiatorOutMin=[]  DifferentiatorOutMax=[]  FilterDiffOutCoefMin=[]  FilterDiffOutCoefMax=[]  ReciprocalOutMin=[]  ReciprocalOutMax=[]  SumDenOutMin=[]  SumDenOutMax=[]  SumNumOutMin=[]  SumNumOutMax=[]  DivideOutMin=[]  DivideOutMax=[]  UdiffTsProdOutMin=[]  UdiffTsProdOutMax=[]  NTsProdOutMin=[]  NTsProdOutMax=[]  UintegralTsProdOutMin=[]  UintegralTsProdOutMax=[]  UngainTsProdOutMin=[]  UngainTsProdOutMax=[]  IntegratorContinuousStateAttributes=''  IntegratorStateMustResolveToSignalObject=off  IntegratorRTWStateStorageClass=Auto  FilterContinuousStateAttributes=''  FilterStateMustResolveToSignalObject=off  FilterRTWStateStorageClass=Auto  ParallelPVariant=InternalParameters  IdealPVariant=Disabled  IVariant=InternalParameters  DVariant=InternalParameters  bVariant=InternalParameters  cVariant=InternalParameters  IntegratorVariant=Discrete  SatVariant=Disabled  AWVariant=Passthrough  PCopyVariant=Disabled  TRVariant=Disabled  FdbkBlocksVariant=Forward  IdealPFdbkVariant=Disabled  SatFdbkVariant=Disabled  DerivativeFilterVariant=ForwardEulerFilter  NVariant=InternalParameters  NCopyVariant=Disabled  FilterICVariant=InternalICsFilter  IntegratorICVariant=InternalICs  ExternalResetVariant=Disabled  TRSumVariant=Passthrough  SumFdbkVariant=Disabled  SumVariant=Sum_PID  TsampFilterVariant=InternalTs  TsampNgainVariant=Passthrough  TsampIntegralVariant=Passthrough  ExternalSaturationOutDataTypeStr=Inherit: Same as second input
      settings: SourceProductBaseCode=SL
  cfblk4 : simulink/Discrete/Transfer Fcn Lead or Lag  PoleZ=0.95  ZeroZ=0.75  ICPrevOutput=0.0  ICPrevInput=0.0  DoSatur=off
      settings: SourceProductBaseCode=SL
  cfblk5 : UnitDelay  SampleTime=-1  HasFrameUpgradeWarning=on
  cfblk6 : Delay
  cfblk7 : Sum  Inputs=-+
  cfblk8 : Abs  SaturateOnIntegerOverflow=off
  cfblk9 : Constant  Value=[810936532.875736]  SampleTime=1
  cfblk2 : Outport
  cfblk14 : Outport  Port=2
  cfblk15 : Outport  Port=3
  wires:
  cfblk8/1 -> cfblk2/1
  cfblk6/1 -> cfblk14/1
  cfblk5/1 -> cfblk8/1
  cfblk4/1 -> cfblk5/1
  cfblk7/1 -> cfblk6/1
  cfblk3/1 -> cfblk10/1(cfblk1)
  cfblk13/1 -> cfblk15/1
  cfblk10/1(cfblk2) -> cfblk11/1(cfblk1)
  cfblk9/1 -> cfblk3/1
  cfblk12/1 -> cfblk10/2(cfblk6)
  cfblk1/1 -> cfblk4/1
  cfblk10/2(cfblk7) -> cfblk11/2(cfblk7), cfblk7/2
  cfblk11/1(cfblk2) -> cfblk7/1
  cfblk11/2(cfblk8) -> cfblk16/1
  cfblk16/1 -> cfblk3/2

== system sampleModel106/cfblk87/cfblk8 ==
  cfblk1 : Inport
  cfblk12 : Inport  Port=2
  cfblk10 : Subsystem
  cfblk11 : Subsystem
  cfblk13 : Delay
  cfblk3 : DiscreteFilter
  cfblk4 : Delay  ShowEnablePort=on
      settings: InputPortMap=u0,e6
  cfblk5 : Sum  Inputs=+
  cfblk6 : MinMax
  cfblk7 : Sum  Inputs=--
  cfblk8 : Signum
  cfblk9 : Constant  Value=[-521409689.533460]  SampleTime=1
  cfblk2 : Outport
  wires:
  cfblk7/1 -> cfblk8/1
  cfblk4/1 -> cfblk11/1(cfblk1)
  cfblk6/1 -> cfblk2/1
  cfblk11/1(cfblk2) -> cfblk10/1(cfblk1)
  cfblk8/1 -> cfblk3/1
  cfblk9/1 -> cfblk6/1
  cfblk3/1 -> cfblk5/1
  cfblk12/1 -> cfblk7/1
  cfblk10/1(cfblk2) -> cfblk7/2
  cfblk1/1 -> cfblk4/1
  cfblk5/1 -> cfblk13/1
  cfblk13/1 -> cfblk4/2

== system sampleModel106/cfblk87/cfblk9 ==
  cfblk1 : Inport
  cfblk16 : Inport  Port=2
  cfblk10 : Constant  Value=[400081457.238042]  SampleTime=1
  cfblk11 : Constant  Value=[961157597.567092]  SampleTime=1
  cfblk12 : Constant  Value=[829536586.607069]  SampleTime=1
  cfblk13 : Subsystem
  cfblk14 : Subsystem
  cfblk15 : Subsystem
  cfblk17 : Delay
  cfblk3 : slpidlib/PID Controller  Controller=PID  Form=Parallel  TimeDomain=Discrete-time  UseExternalTs=off  SampleTime=-1  IntegratorMethod=Forward Euler  FilterMethod=Forward Euler  ControllerParametersSource=internal  P=1  I=1  UseKiTs=off  D=0  N=100  UseFilter=on  TunerSelectOption=Transfer Function Based (PID Tuner App)  InitialConditionSource=internal  InitialConditionForIntegrator=0  InitialConditionForFilter=0  DifferentiatorICPrevScaledInput=0  ExternalReset=none  TrackingMode=off  Kt=1  LimitOutput=off  SatLimitsSource=internal  UpperSaturationLimit=inf  LowerSaturationLimit=-inf  LinearizeAsGain=off  AntiWindupMode=none  Kb=1  POutMin=[]  POutMax=[]  IOutMin=[]  IOutMax=[]  DOutMin=[]  DOutMax=[]  NOutMin=[]  NOutMax=[]  SumOutMin=[]  SumOutMax=[]  SaturationOutMin=[]  SaturationOutMax=[]  PParamMin=[]  PParamMax=[]  IParamMin=[]  IParamMax=[]  DParamMin=[]  DParamMax=[]  NParamMin=[]  NParamMax=[]  KbParamMin=[]  KbParamMax=[]  KtParamMin=[]  KtParamMax=[]  KbOutMin=[]  KbOutMax=[]  KtOutMin=[]  KtOutMax=[]  IntegratorOutMin=[]  IntegratorOutMax=[]  FilterOutMin=[]  FilterOutMax=[]  SumI1OutMin=[]  SumI1OutMax=[]  SumI2OutMin=[]  SumI2OutMax=[]  SumI3OutMin=[]  SumI3OutMax=[]  SumI4OutMin=[]  SumI4OutMax=[]  SumDOutMin=[]  SumDOutMax=[]  DifferentiatorOutMin=[]  DifferentiatorOutMax=[]  FilterDiffOutCoefMin=[]  FilterDiffOutCoefMax=[]  ReciprocalOutMin=[]  ReciprocalOutMax=[]  SumDenOutMin=[]  SumDenOutMax=[]  SumNumOutMin=[]  SumNumOutMax=[]  DivideOutMin=[]  DivideOutMax=[]  UdiffTsProdOutMin=[]  UdiffTsProdOutMax=[]  NTsProdOutMin=[]  NTsProdOutMax=[]  UintegralTsProdOutMin=[]  UintegralTsProdOutMax=[]  UngainTsProdOutMin=[]  UngainTsProdOutMax=[]  IntegratorContinuousStateAttributes=''  IntegratorStateMustResolveToSignalObject=off  IntegratorRTWStateStorageClass=Auto  FilterContinuousStateAttributes=''  FilterStateMustResolveToSignalObject=off  FilterRTWStateStorageClass=Auto  ParallelPVariant=InternalParameters  IdealPVariant=Disabled  IVariant=InternalParameters  DVariant=InternalParameters  IntegratorVariant=Discrete  SatVariant=Disabled  AWVariant=Passthrough  PCopyVariant=Disabled  TRVariant=Disabled  FdbkBlocksVariant=Forward  IdealPFdbkVariant=Disabled  SatFdbkVariant=Disabled  DerivativeFilterVariant=ForwardEulerFilter  NVariant=InternalParameters  NCopyVariant=Disabled  FilterICVariant=InternalICsFilter  IntegratorICVariant=InternalICs  ExternalResetVariant=Disabled  TRSumVariant=Passthrough  SumFdbkVariant=Disabled  SumVariant=Sum_PID  TsampFilterVariant=InternalTs  TsampNgainVariant=Passthrough  TsampIntegralVariant=Passthrough  ExternalSaturationOutDataTypeStr=Inherit: Same as second input  aMode=0
  cfblk4 : DiscreteStateSpace  SampleTime=-1
  cfblk5 : Product
  cfblk6 : Assignment  DiagnosticForDimensions=Warning  IndexOptions=Index vector (dialog)  Indices=1  OutputSizes=1
  cfblk7 : Polyval  Coefs=[ +2.081618890e-019, -1.441693666e-014, +4.719686976e-010, -8.536869453e-006, +1.621573104e-001, -8.087801117e+001 ]
  cfblk8 : simulink/Math Operations/Slider Gain  gain=1  low=0  high=2
  cfblk9 : Constant  Value=[534948626.311637]  SampleTime=1
  cfblk2 : Outport
  wires:
  cfblk9/1 -> cfblk2/1
  cfblk4/1 -> cfblk7/1
  cfblk8/1 -> cfblk3/1
  cfblk1/1 -> cfblk4/1
  cfblk16/1 -> cfblk6/1
  cfblk6/1 -> cfblk15/1(cfblk1)
  cfblk7/1 -> cfblk5/2
  cfblk3/1 -> cfblk15/2(cfblk16)
  cfblk13/1(cfblk2) -> cfblk15/3(cfblk17)
  cfblk11/1 -> cfblk8/1
  cfblk12/1 -> cfblk13/1(cfblk1)
  cfblk5/1 -> cfblk6/2
  cfblk13/2(cfblk8) -> cfblk14/1(cfblk1)
  cfblk10/1 -> cfblk14/2(cfblk8)
  cfblk15/1(cfblk2) -> cfblk17/1
  cfblk17/1 -> cfblk5/1

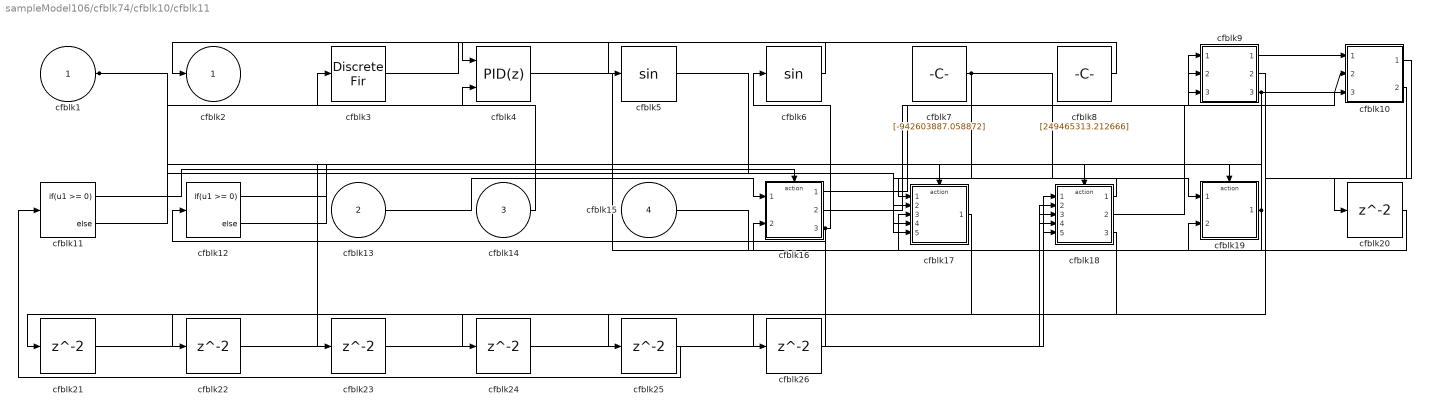
== system sampleModel106/cfblk74/cfblk10/cfblk11 ==
  cfblk1 : Inport
  cfblk13 : Inport  Port=2
  cfblk14 : Inport  Port=3
  cfblk15 : Inport  Port=4
  cfblk10 : Subsystem
  cfblk11 : If  IfExpression=u1 >= 0  SampleTime=1
  cfblk12 : If  IfExpression=u1 >= 0  SampleTime=1
  cfblk16 : Subsystem  TreatAsAtomicUnit=on
  cfblk17 : Subsystem  TreatAsAtomicUnit=on
  cfblk18 : Subsystem  TreatAsAtomicUnit=on
  cfblk19 : Subsystem  TreatAsAtomicUnit=on
  cfblk{20..26} (7 alike) : Delay  SampleTime=1
  cfblk3 : DiscreteFir  SampleTime=1
  cfblk4 : slpidlib/PID Controller (2DOF)  Controller=PID  Form=Parallel  TimeDomain=Discrete-time  UseExternalTs=off  SampleTime=1  IntegratorMethod=Forward Euler  FilterMethod=Forward Euler  ControllerParametersSource=internal  P=1  I=1  UseKiTs=off  D=0  N=100  UseFilter=on  b=1  c=1  TunerSelectOption=Transfer Function Based (PID Tuner App)  InitialConditionSource=internal  InitialConditionForIntegrator=0  InitialConditionForFilter=0  DifferentiatorICPrevScaledInput=0  ExternalReset=none  TrackingMode=off  Kt=1  LimitOutput=off  SatLimitsSource=internal  UpperSaturationLimit=inf  LowerSaturationLimit=-inf  LinearizeAsGain=off  AntiWindupMode=none  Kb=1  POutMin=[]  POutMax=[]  IOutMin=[]  IOutMax=[]  DOutMin=[]  DOutMax=[]  NOutMin=[]  NOutMax=[]  bOutMin=[]  bOutMax=[]  cOutMin=[]  cOutMax=[]  SumOutMin=[]  SumOutMax=[]  SaturationOutMin=[]  SaturationOutMax=[]  PParamMin=[]  PParamMax=[]  IParamMin=[]  IParamMax=[]  DParamMin=[]  DParamMax=[]  NParamMin=[]  NParamMax=[]  bParamMin=[]  bParamMax=[]  cParamMin=[]  cParamMax=[]  KbParamMin=[]  KbParamMax=[]  KtParamMin=[]  KtParamMax=[]  KbOutMin=[]  KbOutMax=[]  KtOutMin=[]  KtOutMax=[]  IntegratorOutMin=[]  IntegratorOutMax=[]  FilterOutMin=[]  FilterOutMax=[]  SumI1OutMin=[]  SumI1OutMax=[]  SumI2OutMin=[]  SumI2OutMax=[]  SumI3OutMin=[]  SumI3OutMax=[]  SumI4OutMin=[]  SumI4OutMax=[]  SumDOutMin=[]  SumDOutMax=[]  Sum1OutMin=[]  Sum1OutMax=[]  Sum2OutMin=[]  Sum2OutMax=[]  Sum3OutMin=[]  Sum3OutMax=[]  DifferentiatorOutMin=[]  DifferentiatorOutMax=[]  FilterDiffOutCoefMin=[]  FilterDiffOutCoefMax=[]  ReciprocalOutMin=[]  ReciprocalOutMax=[]  SumDenOutMin=[]  SumDenOutMax=[]  SumNumOutMin=[]  SumNumOutMax=[]  DivideOutMin=[]  DivideOutMax=[]  UdiffTsProdOutMin=[]  UdiffTsProdOutMax=[]  NTsProdOutMin=[]  NTsProdOutMax=[]  UintegralTsProdOutMin=[]  UintegralTsProdOutMax=[]  UngainTsProdOutMin=[]  UngainTsProdOutMax=[]  IntegratorContinuousStateAttributes=''  IntegratorStateMustResolveToSignalObject=off  IntegratorRTWStateStorageClass=Auto  FilterContinuousStateAttributes=''  FilterStateMustResolveToSignalObject=off  FilterRTWStateStorageClass=Auto  ParallelPVariant=InternalParameters  IdealPVariant=Disabled  IVariant=InternalParameters  DVariant=InternalParameters  bVariant=InternalParameters  cVariant=InternalParameters  IntegratorVariant=Discrete  SatVariant=Disabled  AWVariant=Passthrough  PCopyVariant=Disabled  TRVariant=Disabled  FdbkBlocksVariant=Forward  IdealPFdbkVariant=Disabled  SatFdbkVariant=Disabled  DerivativeFilterVariant=ForwardEulerFilter  NVariant=InternalParameters  NCopyVariant=Disabled  FilterICVariant=InternalICsFilter  IntegratorICVariant=InternalICs  ExternalResetVariant=Disabled  TRSumVariant=Passthrough  SumFdbkVariant=Disabled  SumVariant=Sum_PID  TsampFilterVariant=InternalTs  TsampNgainVariant=Passthrough  TsampIntegralVariant=Passthrough  ExternalSaturationOutDataTypeStr=Inherit: Same as second input
      settings: SourceProductBaseCode=SL
  cfblk5 : Trigonometry
  cfblk6 : Trigonometry
  cfblk7 : Constant  Value=[-942603887.058872]  SampleTime=1
  cfblk8 : Constant  Value=[249465313.212666]  SampleTime=1
  cfblk9 : Subsystem
  cfblk2 : Outport
  wires:
  cfblk14/1 -> cfblk3/1
  cfblk16/1(cfblk2) -> cfblk9/1(cfblk1)
  cfblk16/2(cfblk12) -> cfblk9/2(cfblk8)
  cfblk18/1(cfblk2) -> cfblk17/1(cfblk1)
  cfblk4/1 -> cfblk18/1(cfblk1)
  cfblk6/1 -> cfblk2/1
  cfblk7/1 -> cfblk19/1(cfblk1), cfblk17/4(cfblk15)
  cfblk13/1 -> cfblk16/1(cfblk1)
  cfblk16/3(cfblk13) -> cfblk6/1, cfblk24/1
  cfblk8/1 -> cfblk4/1
  cfblk1/1 -> cfblk4/2, cfblk17/5(cfblk16)
  cfblk19/1(cfblk2) -> cfblk9/3(cfblk9), cfblk17/3(cfblk14)
  cfblk9/1(cfblk2) -> cfblk10/1(cfblk1)
  cfblk15/1 -> cfblk19/2(cfblk7)
  cfblk3/1 -> cfblk5/1
  cfblk9/3(cfblk11) -> cfblk10/2(cfblk12), cfblk23/1
  cfblk18/2(cfblk16) -> cfblk10/3(cfblk13)
  cfblk5/1 -> cfblk17/2(cfblk13)
  cfblk11/1 -> cfblk16/Action
  cfblk11/2 -> cfblk17/Action
  cfblk12/1 -> cfblk18/Action
  cfblk12/2 -> cfblk19/Action
  cfblk10/1(cfblk2) -> cfblk20/1
  cfblk20/1 -> cfblk16/2(cfblk11)
  cfblk10/2(cfblk14) -> cfblk21/1
  cfblk21/1 -> cfblk18/3(cfblk13)
  cfblk9/2(cfblk10) -> cfblk22/1
  cfblk22/1 -> cfblk18/2(cfblk12)
  cfblk23/1 -> cfblk18/4(cfblk14)
  cfblk24/1 -> cfblk18/5(cfblk15)
  cfblk17/1(cfblk2) -> cfblk25/1
  cfblk25/1 -> cfblk11/1
  cfblk18/3(cfblk17) -> cfblk26/1
  cfblk26/1 -> cfblk12/1

== system sampleModel106/cfblk74/cfblk11/cfblk6 ==
  cfblk1 : Inport
  cfblk12 : Inport  Port=2
  cfblk13 : Inport  Port=3
  cfblk14 : Inport  Port=4
  cfblk15 : Inport  Port=5
  cfblk10 : Subsystem
  cfblk11 : If  IfExpression=u1 >= 0  SampleTime=1
  cfblk17 : Subsystem  TreatAsAtomicUnit=on
  cfblk18 : Subsystem  TreatAsAtomicUnit=on
  cfblk{19..22} (4 alike) : Delay  SampleTime=1
  cfblk3 : Polyval  Coefs=[ +2.081618890e-019, -1.441693666e-014, +4.719686976e-010, -8.536869453e-006, +1.621573104e-001, -8.087801117e+001 ]
  cfblk4 : Product  Inputs=*
  cfblk5 : Constant  Value=[362525032.245355]  SampleTime=1
  cfblk6 : Subsystem
  cfblk7 : Subsystem
  cfblk8 : Subsystem
  cfblk9 : Subsystem
  cfblk2 : Outport
  cfblk16 : Outport  Port=2
  wires:
  cfblk10/1(cfblk2) -> cfblk7/1(cfblk1)
  cfblk13/1 -> cfblk4/1
  cfblk9/1(cfblk2) -> cfblk18/1(cfblk1)
  cfblk12/1 -> cfblk16/1
  cfblk9/2(cfblk10) -> cfblk10/1(cfblk1)
  cfblk7/1(cfblk2) -> cfblk6/1(cfblk1)
  cfblk14/1 -> cfblk2/1
  cfblk7/2(cfblk11) -> cfblk6/2(cfblk13)
  cfblk1/1 -> cfblk3/1
  cfblk18/2(cfblk9) -> cfblk6/3(cfblk14)
  cfblk6/1(cfblk2) -> cfblk8/1(cfblk1)
  cfblk5/1 -> cfblk8/2(cfblk6)
  cfblk10/2(cfblk16) -> cfblk17/1(cfblk1)
  cfblk8/2(cfblk7) -> cfblk17/2(cfblk13)
  cfblk9/3(cfblk11) -> cfblk11/1
  cfblk15/1 -> cfblk10/4(cfblk14)
  cfblk6/2(cfblk15) -> cfblk17/3(cfblk14)
  cfblk4/1 -> cfblk10/5(cfblk15)
  cfblk11/1 -> cfblk17/Action
  cfblk11/2 -> cfblk18/Action
  cfblk8/1(cfblk2) -> cfblk19/1
  cfblk19/1 -> cfblk10/3(cfblk13)
  cfblk17/1(cfblk2) -> cfblk20/1
  cfblk20/1 -> cfblk7/2(cfblk10)
  cfblk17/2(cfblk15) -> cfblk21/1
  cfblk21/1 -> cfblk10/2(cfblk12)
  cfblk18/1(cfblk2) -> cfblk22/1
  cfblk22/1 -> cfblk9/1(cfblk1)

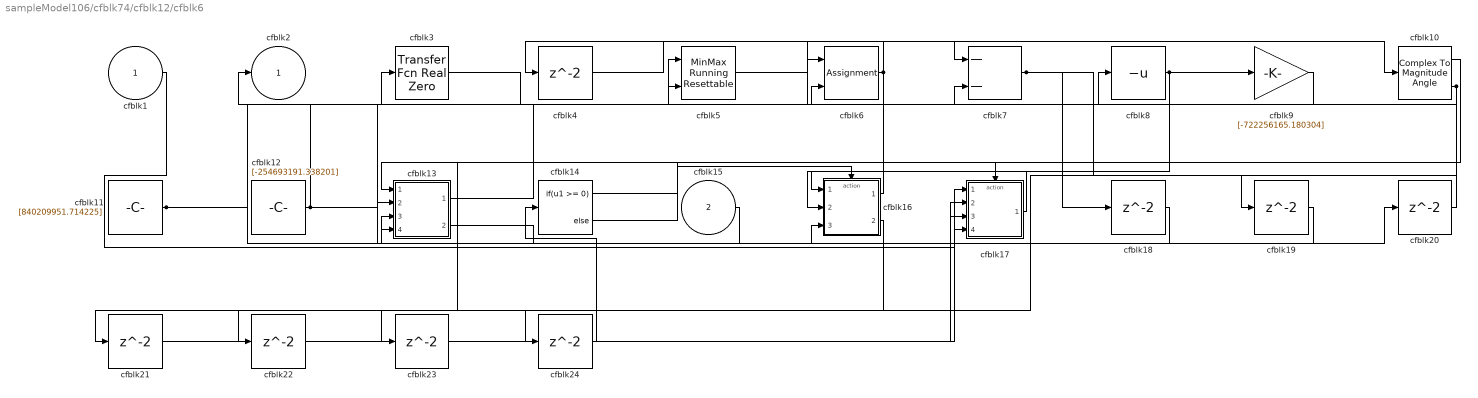
== system sampleModel106/cfblk74/cfblk12/cfblk6 ==
  cfblk1 : Inport
  cfblk15 : Inport  Port=2
  cfblk10 : ComplexToMagnitudeAngle
  cfblk11 : Constant  Value=[840209951.714225]  SampleTime=1
  cfblk12 : Constant  Value=[-254693191.338201]  SampleTime=1
  cfblk13 : Subsystem
  cfblk14 : If  IfExpression=u1 >= 0  SampleTime=1
  cfblk16 : Subsystem  TreatAsAtomicUnit=on
  cfblk17 : Subsystem  TreatAsAtomicUnit=on
  cfblk{4,18..24} (8 alike) : Delay  SampleTime=1
  cfblk3 : simulink/Discrete/Transfer Fcn Real Zero  ZeroZ=0.75  ICPrevInput=0.0  DoSatur=off
      settings: SourceProductBaseCode=SL
  cfblk5 : simulink/Math Operations/MinMax Running Resettable  Function=min  vinit=0.0
  cfblk6 : Assignment  DiagnosticForDimensions=Warning  IndexOptions=Index vector (dialog)  Indices=1  OutputSizes=1
  cfblk7 : Sum  Inputs=--
  cfblk8 : UnaryMinus
  cfblk9 : Gain  Gain=[-722256165.180304]
  cfblk2 : Outport
  wires:
  cfblk17/1(cfblk2) -> cfblk16/1(cfblk1)
  cfblk6/1 -> cfblk4/1, cfblk23/1
  cfblk10/1 -> cfblk13/1(cfblk1)
  cfblk8/1 -> cfblk9/1, cfblk16/2(cfblk8)
  cfblk13/1(cfblk2) -> cfblk5/1
  cfblk16/1(cfblk2) -> cfblk6/2
  cfblk3/1 -> cfblk5/2
  cfblk11/1 -> cfblk3/1, cfblk16/3(cfblk9)
  cfblk1/1 -> cfblk17/1(cfblk1)
  cfblk5/1 -> cfblk7/1
  cfblk9/1 -> cfblk7/2
  cfblk7/1 -> cfblk18/1, cfblk19/1
  cfblk4/1 -> cfblk10/1
  cfblk15/1 -> cfblk13/3(cfblk11)
  cfblk10/2 -> cfblk21/1, cfblk22/1
  cfblk12/1 -> cfblk2/1, cfblk8/1
  cfblk14/1 -> cfblk16/Action
  cfblk14/2 -> cfblk17/Action
  cfblk18/1 -> cfblk13/2(cfblk10)
  cfblk19/1 -> cfblk13/4(cfblk12)
  cfblk13/2(cfblk13) -> cfblk20/1
  cfblk20/1 -> cfblk6/1
  cfblk21/1 -> cfblk17/2(cfblk15)
  cfblk22/1 -> cfblk17/4(cfblk17)
  cfblk23/1 -> cfblk17/3(cfblk16)
  cfblk16/2(cfblk10) -> cfblk24/1
  cfblk24/1 -> cfblk14/1

== system sampleModel106/cfblk74/cfblk12/cfblk7 ==
  cfblk1 : Inport
  cfblk3 : simulink/Discrete/Transfer Fcn Real Zero  ZeroZ=0.75  ICPrevInput=0.0  DoSatur=off
      settings: SourceProductBaseCode=SL
  cfblk4 : Product  Inputs=*
  cfblk5 : Polyval  Coefs=[ +2.081618890e-019, -1.441693666e-014, +4.719686976e-010, -8.536869453e-006, +1.621573104e-001, -8.087801117e+001 ]
  cfblk6 : Rounding
  cfblk7 : Subsystem
  cfblk8 : Delay  SampleTime=1
  cfblk9 : Delay  SampleTime=1
  cfblk2 : Outport
  wires:
  cfblk4/1 -> cfblk5/1
  cfblk1/1 -> cfblk6/1
  cfblk5/1 -> cfblk8/1, cfblk9/1
  cfblk7/1(cfblk2) -> cfblk4/1
  cfblk7/2(cfblk15) -> cfblk2/1
  cfblk6/1 -> cfblk3/1
  cfblk3/1 -> cfblk7/2(cfblk13)
  cfblk8/1 -> cfblk7/1(cfblk1)
  cfblk9/1 -> cfblk7/3(cfblk14)

== system sampleModel106/cfblk74/cfblk12/cfblk8 ==
  cfblk1 : Inport
  cfblk9 : Inport  Port=2
  cfblk10 : Inport  Port=3
  cfblk11 : Inport  Port=4
  cfblk14 : Delay  SampleTime=1
  cfblk3 : simulink/Discrete/Transfer Fcn Real Zero  ZeroZ=0.75  ICPrevInput=0.0  DoSatur=off
      settings: SourceProductBaseCode=SL
  cfblk4 : DiscreteFilter  SampleTime=1
  cfblk5 : DotProduct  OutDataTypeStr=Inherit: Inherit via internal rule
  cfblk6 : Gain  Gain=[867715043.927985]
  cfblk7 : Reshape
  cfblk8 : Subsystem
  cfblk2 : Outport
  cfblk12 : Outport  Port=2
  cfblk13 : Outport  Port=3
  wires:
  cfblk7/1 -> cfblk8/1(cfblk1)
  cfblk9/1 -> cfblk4/1
  cfblk4/1 -> cfblk6/1
  cfblk10/1 -> cfblk2/1
  cfblk11/1 -> cfblk3/1
  cfblk6/1 -> cfblk5/1
  cfblk3/1 -> cfblk13/1
  cfblk1/1 -> cfblk12/1
  cfblk5/1 -> cfblk7/1
  cfblk8/1(cfblk2) -> cfblk14/1
  cfblk14/1 -> cfblk5/2
